simulink model "controllerJohnny"  (R2025b)
settings: Solver=ode45  StartTime=0.0  StopTime=15  RelTol=1e-3
values from neighbouring files (symbols this model uses):
  Ts = 0.01    [main.m]
settings Model: Creator=User  LastModifiedBy=User

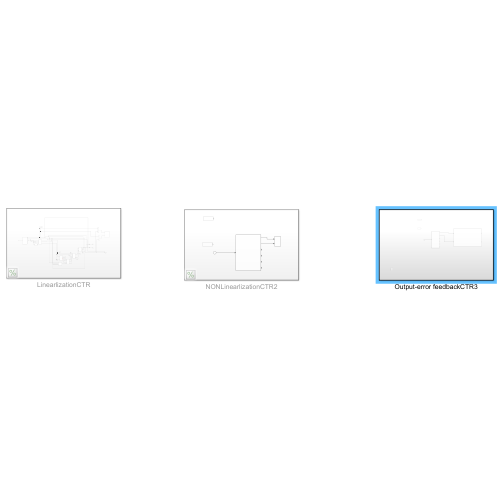
[thumbnail: Simulink's stored preview of the top-level diagram]
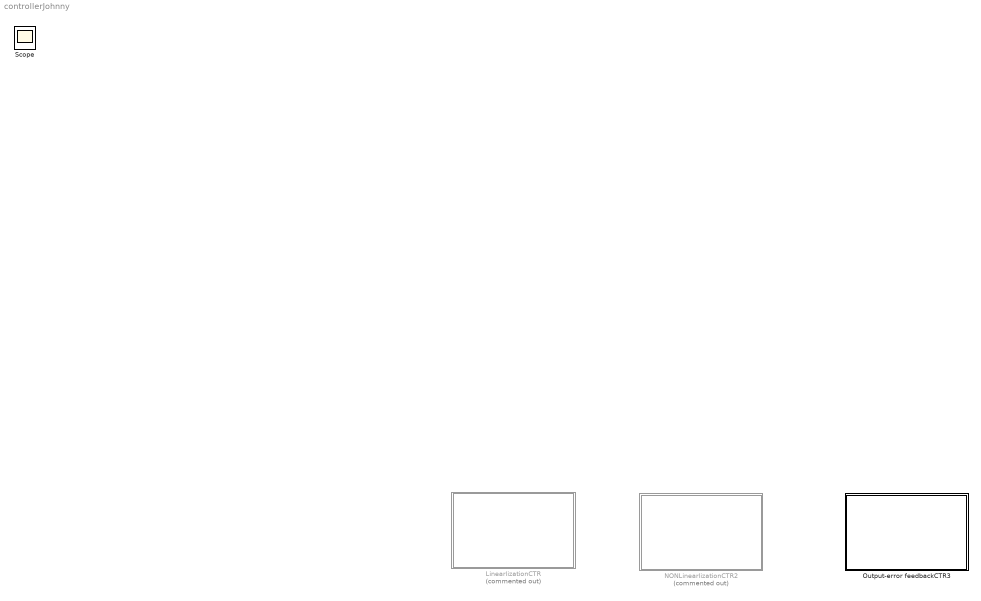
== system controllerJohnny ==
  LinearlizationCTR : Subsystem  Commented=on
  NONLinearlizationCTR2 : Subsystem  Commented=on
  Output-error feedbackCTR3 : Subsystem
  Scope : Scope
      settings: DataLoggingVariableName=ScopeData15

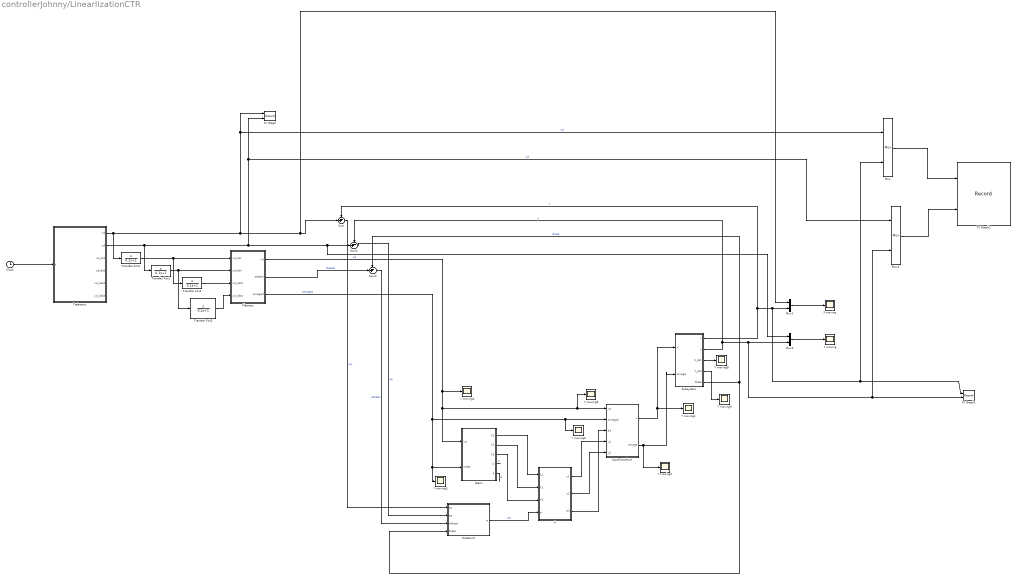
== system controllerJohnny/LinearlizationCTR ==
  Clock : Clock
  Flatness : MATLAB Function  TreatAsAtomicUnit=on
  Gians : MATLAB Function  TreatAsAtomicUnit=on
  InputTransform : MATLAB Function  TreatAsAtomicUnit=on
  Mux{,1,3..4} (4 alike) : Mux  Inputs=2
  Rotation1 : MATLAB Function  TreatAsAtomicUnit=on
  Subsystem : Subsystem
  Sum : Sum  Inputs=-+|
  Sum1 : Sum  Inputs=-+|
  Sum2 : Sum  Inputs=-+|
  Trajectory : MATLAB Function  TreatAsAtomicUnit=on
  Transfer Fcn{1..4} (4 alike) : TransferFcn  Numerator=[1 0]  Denominator=[0.1 1]
  U : MATLAB Function  TreatAsAtomicUnit=on
  X moving : Scope
      settings: ActiveDisplayYMinimum=-7.5707248352770318  ActiveDisplayYMaximum=6.89936023828367  DataLoggingVariableName=ScopeData2
  XY Graph : Record  NumPorts=2.0  FileSettingsInternal="{\"entries\":[{\"content\":{\"excelSettings\":{\"content\":{},\"type\":\"Streamout.ExcelSettings\"},\"parquetSettings\":{\"content\":{},\"type\":\"Streamout.ParquetSettings\"}},\"type\":\"Streamout.FileSettingStorage\",\"uuid\":\"\"}],\"packageUris\":[\"http:\\/\\/schema.mathworks.com\\/mf0\\/streamout_blocks\\/R2020a\"],\"version\":\"1.0\"}"  FrameSettings=[0, 0]  Layout=[1 1]  SignalsInternal="{\"entries\":[{\"content\":{},\"type\":\"RecordBlkView.InputSignals\",\"uuid\":\"\"}],\"packageUris\":[\"http:\\/\\/schema.mathworks.com\\/mf0\\/streamout_blocks\\/R2020a\"],\"version\":\"1.0\"}"  VisualizationBindings="{\"xyplotplugin\":{\"info\":[{\"series\":[],\"subplotID\":1}]}}"  CompatibilityTag=XY
  XY Graph1 : Record  NumPorts=2.0  FileSettingsInternal="{\"entries\":[{\"content\":{\"excelSettings\":{\"content\":{},\"type\":\"Streamout.ExcelSettings\"},\"parquetSettings\":{\"content\":{},\"type\":\"Streamout.ParquetSettings\"}},\"type\":\"Streamout.FileSettingStorage\",\"uuid\":\"\"}],\"packageUris\":[\"http:\\/\\/schema.mathworks.com\\/mf0\\/streamout_blocks\\/R2020a\"],\"version\":\"1.0\"}"  FrameSettings=[0, 0]  Layout=[1 1]  SignalsInternal="{\"entries\":[{\"content\":{},\"type\":\"RecordBlkView.InputSignals\",\"uuid\":\"\"}],\"packageUris\":[\"http:\\/\\/schema.mathworks.com\\/mf0\\/streamout_blocks\\/R2020a\"],\"version\":\"1.0\"}"  VisualizationBindings="{\"xyplotplugin\":{\"info\":[{\"series\":[],\"subplotID\":1}]}}"  CompatibilityTag=XY
  XY Graph2 : Record  NumPorts=2.0  FileSettingsInternal="{\"entries\":[{\"content\":{\"excelSettings\":{\"content\":{},\"type\":\"Streamout.ExcelSettings\"},\"parquetSettings\":{\"content\":{},\"type\":\"Streamout.ParquetSettings\"}},\"type\":\"Streamout.FileSettingStorage\",\"uuid\":\"\"}],\"packageUris\":[\"http:\\/\\/schema.mathworks.com\\/mf0\\/streamout_blocks\\/R2020a\"],\"version\":\"1.0\"}"  FrameSettings=[0, 0]  Layout=[1 1]  SignalsInternal="{\"entries\":[{\"content\":{\"signals\":[{\"content\":{\"blockPath\":[],\"dimensions\":[1],\"domain\":\"\",\"lineColor\":\"#ff6929\",\"lineWidth\":2,\"port\":1,\"signalID\":1,\"signalName\":\"Mux\"},\"type\":\"RecordBlkView.Signal\",\"uuid\":\"\"},{\"content\":{\"blockPath\":[],\"dimensions\":[1],\"domain\":\"\",\"lineColor\":\"#b746ff\",\"lineWidth\":2,\"port\":2,\"signalID\":2,\"signalName\":\"Mux4\"},\"type\":\"RecordBlkView.Signal\",\"uuid\":\"\"}]},\"type\":\"RecordBlkView.InputSignals\",\"uuid\":\"\"}],\"packageUris\":[\"http:\\/\\/schema.mathworks.com\\/mf0\\/streamout_blocks\\/R2020a\"],\"version\":\"1.0\"}"  VisualizationBindings="{\"xyplotplugin\":{\"info\":[{\"series\":[],\"subplotID\":1}]}}"  CompatibilityTag=XY
  Y moving{,1..6,8..9} (9 alike) : Scope
      Y moving settings: ActiveDisplayYMinimum=-5.0263813296916764  ActiveDisplayYMaximum=5.2374840982446349  DataLoggingVariableName=ScopeData3
      Y moving1 settings: ActiveDisplayYMinimum=-34.324914712581226  ActiveDisplayYMaximum=308.9242324132311  DataLoggingVariableName=ScopeData4
      Y moving2 settings: ActiveDisplayYMinimum=-1.6157130196688239E+7  ActiveDisplayYMaximum=1.4491472238781191E+7  DataLoggingVariableName=ScopeData5
      Y moving3 settings: ActiveDisplayYMinimum=4.999999999999944  ActiveDisplayYMaximum=5.0000000000000542  DataLoggingVariableName=ScopeData6
      Y moving4 settings: ActiveDisplayYMinimum=9.9999999999999982  ActiveDisplayYMaximum=10.000000000000002  DataLoggingVariableName=ScopeData7
      Y moving5 settings: ActiveDisplayYMinimum=0.99999999999999978  ActiveDisplayYMaximum=1  DataLoggingVariableName=ScopeData8
      Y moving6 settings: ActiveDisplayYMinimum=0.4  ActiveDisplayYMaximum=0.60000000000000009  DataLoggingVariableName=ScopeData9
      Y moving8 settings: ActiveDisplayYMinimum=-4.8047106790322678  ActiveDisplayYMaximum=12.533856742114697  DataLoggingVariableName=ScopeData11
      Y moving9 settings: ActiveDisplayYMinimum=-3.6998487914435718  ActiveDisplayYMaximum=4.6099967599268465  DataLoggingVariableName=ScopeData12
  wires:
  Subsystem/1(x) -> Mux/2, XY Graph1/1, Mux1/2, Sum/1  "x"
  Subsystem/5(theta) -> Rotation1/4(theta), Sum2/1  "theta"
  Trajectory/1(xd) -> Transfer Fcn4/1, Mux/1, XY Graph/1, Mux1/1, Sum/2  "xd"
  Flatness/3(omegad) -> Y moving3/1, Gians/2(wdes), Y moving6/1, InputTransform/2(omegad)  "omegad"
  Sum2/1 -> Rotation1/3(etheta)  "etheta"
  Gians/2(k2) -> U/2(k2)
  Sum/1 -> Rotation1/1(ex)  "ex"
  InputTransform/2(omega) -> Y moving2/1, Subsystem/2(omega)
  U/3(e3) -> InputTransform/3(e3)
  InputTransform/1(v) -> Subsystem/1(V), Y moving1/1
  Rotation1/1(e) -> U/4(e)  "ew"
  Gians/3(k3) -> U/3(k3)
  Gians/1(k1) -> U/1(k1)
  Flatness/1(vd) -> Y moving4/1, Gians/1(vd), Y moving5/1, InputTransform/1(vd)  "vd"
  Mux3/1 -> Y moving/1
  Subsystem/4(Y_dot) -> Y moving9/1
  Flatness/2(thetad) -> Sum2/2  "thetad"
  Subsystem/2(y) -> Mux4/2, XY Graph1/2, Mux3/2, Sum1/1  "y"
  Mux1/1 -> X moving/1
  U/1(u1) -> InputTransform/4(u1)
  Clock/1 -> Trajectory/1(t)
  Subsystem/3(X_dot) -> Y moving8/1
  U/2(u2) -> InputTransform/5(u2)
  Sum1/1 -> Rotation1/2(ey)  "ey"
  Mux4/1 -> XY Graph2/2
  Mux/1 -> XY Graph2/1
  Trajectory/2(yd) -> Transfer Fcn1/1, Mux4/1, XY Graph/2, Mux3/1, Sum1/2  "yd"
  Transfer Fcn4/1 -> Transfer Fcn2/1, Flatness/1(xd_dot)
  Transfer Fcn1/1 -> Flatness/2(yd_dot), Transfer Fcn3/1
  Transfer Fcn2/1 -> Flatness/3(xd_ddot)
  Transfer Fcn3/1 -> Flatness/4(yd_ddot)
  Gians/5(a) -> ?  "a"
  Gians/4(xi) -> ?  "xi"

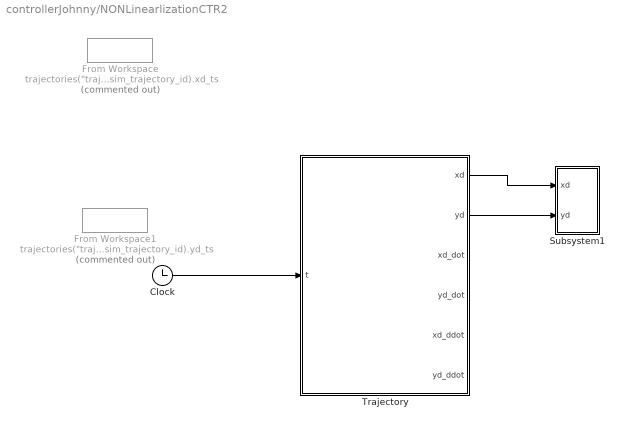
== system controllerJohnny/NONLinearlizationCTR2 ==
  Clock : Clock
  From Workspace : FromWorkspace  Commented=on  VariableName="trajectories(\"trajectory\"+sim_trajectory_id).xd_ts"  SampleTime=Ts  OutputAfterFinalValue=Holding final value
  From Workspace1 : FromWorkspace  Commented=on  VariableName="trajectories(\"trajectory\"+sim_trajectory_id).yd_ts"  SampleTime=Ts  OutputAfterFinalValue=Holding final value
  Subsystem1 : Subsystem
  Trajectory : MATLAB Function  TreatAsAtomicUnit=on
  wires:
  Clock/1 -> Trajectory/1(t)
  Trajectory/2(yd) -> Subsystem1/2(yd)
  Trajectory/1(xd) -> Subsystem1/1(xd)

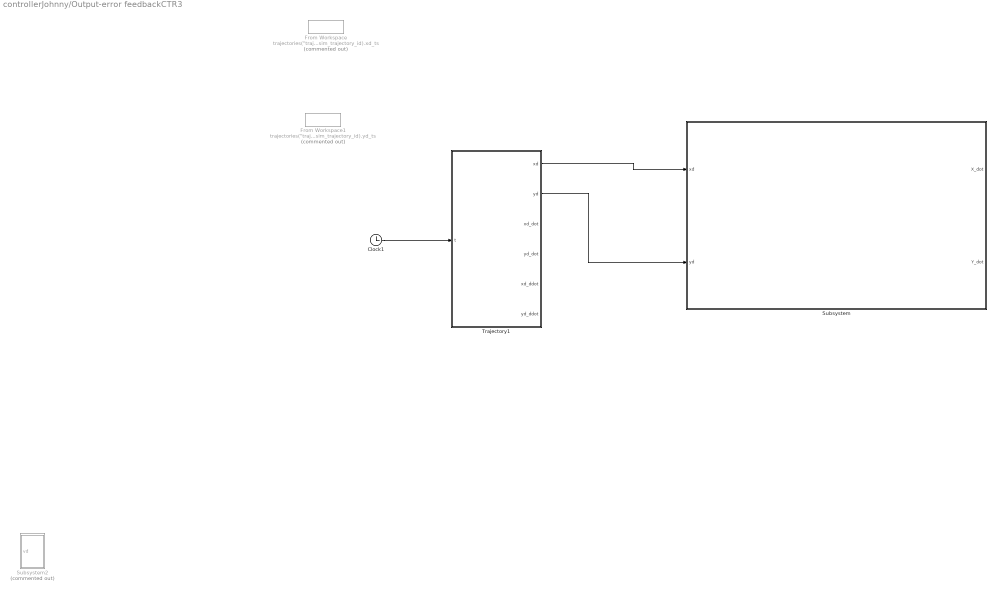
== system controllerJohnny/Output-error feedbackCTR3 ==
  Clock1 : Clock
  From Workspace : FromWorkspace  Commented=on  VariableName="trajectories(\"trajectory\"+sim_trajectory_id).xd_ts"  SampleTime=Ts  OutputAfterFinalValue=Holding final value
  From Workspace1 : FromWorkspace  Commented=on  VariableName="trajectories(\"trajectory\"+sim_trajectory_id).yd_ts"  SampleTime=Ts  OutputAfterFinalValue=Holding final value
  Subsystem : Subsystem
  Subsystem2 : Subsystem  Commented=on
  Trajectory1 : MATLAB Function  TreatAsAtomicUnit=on
  wires:
  Clock1/1 -> Trajectory1/1(t)
  Trajectory1/1(xd) -> Subsystem/1(xd)
  Trajectory1/2(yd) -> Subsystem/2(yd)

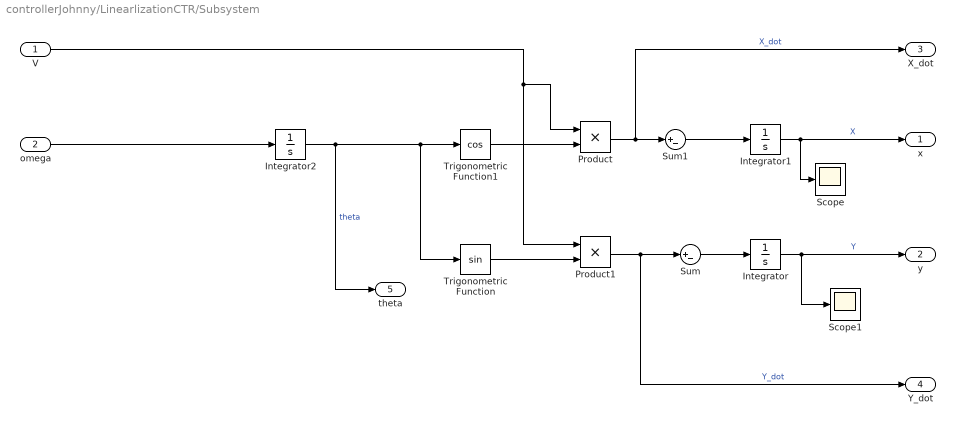
== system controllerJohnny/LinearlizationCTR/Subsystem ==
  V : Inport
  omega : Inport  Port=2
  Integrator : Integrator
  Integrator1 : Integrator
  Integrator2 : Integrator
  Product : Product
  Product1 : Product
  Scope : Scope
      settings: ActiveDisplayYMinimum=-0.63591257102151144  ActiveDisplayYMaximum=2.8001536498931303
  Scope1 : Scope
      settings: ActiveDisplayYMinimum=-1.1667967618896729  ActiveDisplayYMaximum=3.6680934698341847
  Sum : Sum  Inputs=|+-
  Sum1 : Sum  Inputs=|+-
  Trigonometric Function : Trigonometry
  Trigonometric Function1 : Trigonometry  Operator=cos
  x : Outport
  y : Outport  Port=2
  X_dot : Outport  Port=3
  Y_dot : Outport  Port=4
  theta : Outport  Port=5
  wires:
  Integrator/1 -> Scope1/1, y/1  "Y"
  Integrator2/1 -> theta/1, Trigonometric Function/1, Trigonometric Function1/1  "theta"
  Sum/1 -> Integrator/1
  V/1 -> Product/1, Product1/1
  Trigonometric Function1/1 -> Product/2
  Sum1/1 -> Integrator1/1
  Product/1 -> X_dot/1, Sum1/1  "X_dot"
  Integrator1/1 -> Scope/1, x/1  "X"
  Product1/1 -> Y_dot/1, Sum/1  "Y_dot"
  Trigonometric Function/1 -> Product1/2
  omega/1 -> Integrator2/1

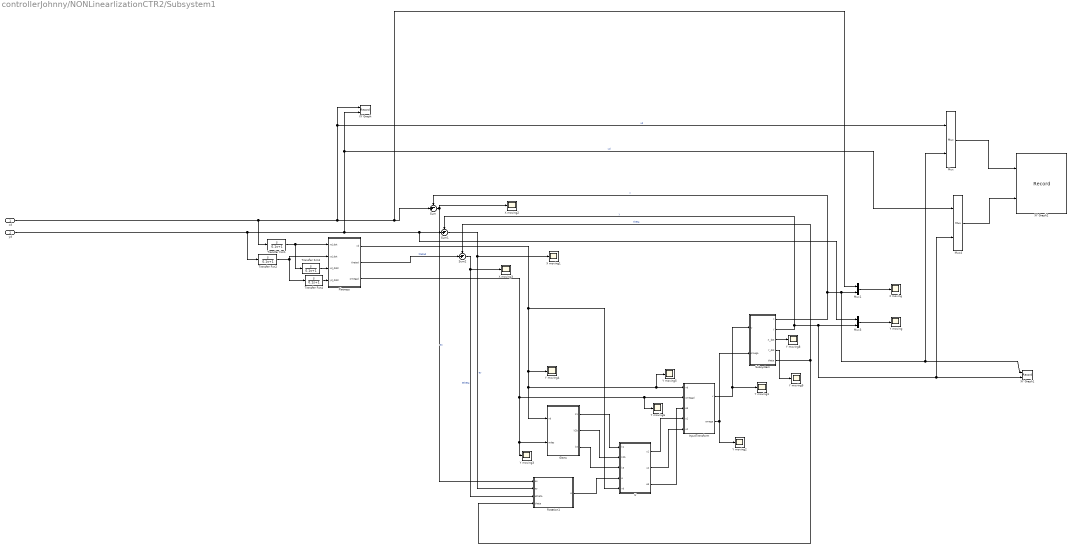
== system controllerJohnny/NONLinearlizationCTR2/Subsystem1 ==
  xd : Inport
  yd : Inport  Port=2
  Flatness : MATLAB Function  TreatAsAtomicUnit=on
  Gians : MATLAB Function  TreatAsAtomicUnit=on
  InputTransform : MATLAB Function  TreatAsAtomicUnit=on
  Mux{,1,3..4} (4 alike) : Mux  Inputs=2
  Rotation1 : MATLAB Function  TreatAsAtomicUnit=on
  Subsystem : Subsystem
  Sum : Sum  Inputs=-+|
  Sum1 : Sum  Inputs=-+|
  Sum2 : Sum  Inputs=-+|
  Transfer Fcn{1..4} (4 alike) : TransferFcn  Numerator=[1 0]  Denominator=[0.1 1]
  U : MATLAB Function  TreatAsAtomicUnit=on
  X moving{,1..3} (4 alike) : Scope
      X moving settings: ActiveDisplayYMinimum=-363.26549927941852  ActiveDisplayYMaximum=-359.6142263759865  DataLoggingVariableName=ScopeData2
      X moving1 settings: ActiveDisplayYMinimum=-1.8783922722321265  ActiveDisplayYMaximum=1.6589955287132554  DataLoggingVariableName=ScopeData10
      X moving2 settings: ActiveDisplayYMinimum=-3.0823097685833254  ActiveDisplayYMaximum=2.0935592914317827  DataLoggingVariableName=ScopeData13
      X moving3 settings: ActiveDisplayYMinimum=-3.3439097799700566  ActiveDisplayYMaximum=4.453783260307695  DataLoggingVariableName=ScopeData14
  XY Graph : Record  NumPorts=2.0  FileSettingsInternal="{\"entries\":[{\"content\":{\"excelSettings\":{\"content\":{},\"type\":\"Streamout.ExcelSettings\"},\"parquetSettings\":{\"content\":{},\"type\":\"Streamout.ParquetSettings\"}},\"type\":\"Streamout.FileSettingStorage\",\"uuid\":\"\"}],\"packageUris\":[\"http:\\/\\/schema.mathworks.com\\/mf0\\/streamout_blocks\\/R2020a\"],\"version\":\"1.0\"}"  FrameSettings=[0, 0]  Layout=[1 1]  SignalsInternal="{\"entries\":[{\"content\":{\"signals\":[{\"content\":{\"blockPath\":[],\"dimensions\":[1],\"domain\":\"\",\"lineColor\":\"#ff13a6\",\"lineWidth\":2,\"port\":1,\"signalID\":1,\"signalName\":\"xd\"},\"type\":\"RecordBlkView.Signal\",\"uuid\":\"\"},{\"content\":{\"blockPath\":[],\"dimensions\":[1],\"domain\":\"\",\"lineColor\":\"#fe330a\",\"lineWidth\":2,\"port\":2,\"signalID\":2,\"signalName\":\"yd\"},\"type\":\"RecordBlkView.Signal\",\"uuid\":\"\"}]},\"type\":\"RecordBlkView.InputSignals\",\"uuid\":\"\"}],\"packageUris\":[\"http:\\/\\/schema.mathworks.com\\/mf0\\/streamout_blocks\\/R2020a\"],\"version\":\"1.0\"}"  VisualizationBindings="{\"xyplotplugin\":{\"info\":[{\"series\":[],\"subplotID\":1}]}}"  CompatibilityTag=XY
  XY Graph1 : Record  NumPorts=2.0  FileSettingsInternal="{\"entries\":[{\"content\":{\"excelSettings\":{\"content\":{},\"type\":\"Streamout.ExcelSettings\"},\"parquetSettings\":{\"content\":{},\"type\":\"Streamout.ParquetSettings\"}},\"type\":\"Streamout.FileSettingStorage\",\"uuid\":\"\"}],\"packageUris\":[\"http:\\/\\/schema.mathworks.com\\/mf0\\/streamout_blocks\\/R2020a\"],\"version\":\"1.0\"}"  FrameSettings=[0, 0]  Layout=[1 1]  SignalsInternal="{\"entries\":[{\"content\":{\"signals\":[{\"content\":{\"blockPath\":[],\"dimensions\":[1],\"domain\":\"\",\"lineColor\":\"#22b573\",\"lineWidth\":2,\"port\":1,\"signalID\":1,\"signalName\":\"x\"},\"type\":\"RecordBlkView.Signal\",\"uuid\":\"\"},{\"content\":{\"blockPath\":[],\"dimensions\":[1],\"domain\":\"\",\"lineColor\":\"#0072bd\",\"lineWidth\":2,\"port\":2,\"signalID\":2,\"signalName\":\"y\"},\"type\":\"RecordBlkView.Signal\",\"uuid\":\"\"}]},\"type\":\"RecordBlkView.InputSignals\",\"uuid\":\"\"}],\"packageUris\":[\"http:\\/\\/schema.mathworks.com\\/mf0\\/streamout_blocks\\/R2020a\"],\"version\":\"1.0\"}"  VisualizationBindings="{\"xyplotplugin\":{\"info\":[{\"series\":[],\"subplotID\":1}]}}"  CompatibilityTag=XY
  XY Graph2 : Record  NumPorts=2.0  FileSettingsInternal="{\"entries\":[{\"content\":{\"excelSettings\":{\"content\":{},\"type\":\"Streamout.ExcelSettings\"},\"parquetSettings\":{\"content\":{},\"type\":\"Streamout.ParquetSettings\"}},\"type\":\"Streamout.FileSettingStorage\",\"uuid\":\"\"}],\"packageUris\":[\"http:\\/\\/schema.mathworks.com\\/mf0\\/streamout_blocks\\/R2020a\"],\"version\":\"1.0\"}"  FrameSettings=[0, 0]  Layout=[1 1]  SignalsInternal="{\"entries\":[{\"content\":{\"signals\":[{\"content\":{\"blockPath\":[],\"dimensions\":[2],\"domain\":\"\",\"hasChildren\":true,\"lineColor\":\"#64d413\",\"lineWidth\":2,\"port\":1,\"signalID\":1,\"signalName\":\"Mux\"},\"type\":\"RecordBlkView.Signal\",\"uuid\":\"\"},{\"content\":{\"blockPath\":[],\"channel\":[1],\"dimensions\":[2],\"domain\":\"\",\"lineColor\":\"#edb120\",\"lineWidth\":2,\"parentID\":1,\"port\":1,\"signalID\":2,\"signalName\":\"Mux\"},\"type\":\"RecordBlkView.Signal\",\"uuid\":\"\"},{\"content\":{\"blockPath\":[],\"channel\":[2],\"dimensions\":[2],\"domain\":\"\",\"lineColor\":\"#4dbeee\",\"lineWidth\":2,\"parentID\":1,\"port\":1,\"signalID\":3,\"signalName\":\"Mux\"},\"type\":\"RecordBlkView.Signal\",\"uuid\":\"\"},{\"content\":{\"blockPath\":[],\"dimensions\":[2],\"domain\":\"\",\"hasChildren\":true,\"lineColor\":\"#fe330a\",\"lineWidth\":2,\"port\":2,\"signalID\":4,\"signalName\":\"Mux4\"},\"type\":\"RecordBlkView.Signal\",\"uuid\":\"\"},{\"content\":{\"blockPath\":[],\"channel\":[1],\"dimensions\":[2],\"domain\":\"\",\"lineColor\":\"#77ac30\",\"lineWidth\":2,\"parentID\":4,\"port\":2,\"signalID\":5,\"signalName\":\"Mux4\"},\"type\":\"RecordBlkView.Signal\",\"uuid\":\"\"},{\"content\":{\"blockPath\":[],\"channel\":[2],\"dimensions\":[2],\"domain\":\"\",\"lineColor\":\"#a2142f\",\"lineWidth\":2,\"parentID\":4,\"port\":2,\"signalID\":6,\"signalName\":\"Mux4\"},\"type\":\"RecordBlkView.Signal\",\"uuid\":\"\"}]},\"type\":\"RecordBlkView.InputSignals\",\"uuid\":\"\"}],\"packageUris\":[\"http:\\/\\/schema.mathworks.com\\/mf0\\/streamout_blocks\\/R2020a\"],\"version\":\"1.0\"}"  VisualizationBindings="{\"xyplotplugin\":{\"info\":[{\"series\":[],\"subplotID\":1}]}}"  CompatibilityTag=XY
  Y moving{,1..6,8..9} (9 alike) : Scope
      Y moving settings: ActiveDisplayYMinimum=-7.4999627279123162  ActiveDisplayYMaximum=7.4999958513257434  DataLoggingVariableName=ScopeData3
      Y moving1 settings: ActiveDisplayYMinimum=-34.324914712581226  ActiveDisplayYMaximum=308.9242324132311  DataLoggingVariableName=ScopeData4
      Y moving2 settings: ActiveDisplayYMinimum=-1.6157130196688239E+7  ActiveDisplayYMaximum=1.4491472238781191E+7  DataLoggingVariableName=ScopeData5
      Y moving3 settings: ActiveDisplayYMinimum=4.999999999999944  ActiveDisplayYMaximum=5.0000000000000542  DataLoggingVariableName=ScopeData6
      Y moving4 settings: ActiveDisplayYMinimum=9.9999999999999982  ActiveDisplayYMaximum=10.000000000000002  DataLoggingVariableName=ScopeData7
      Y moving5 settings: ActiveDisplayYMinimum=0.99999999999999978  ActiveDisplayYMaximum=1  DataLoggingVariableName=ScopeData8
      Y moving6 settings: ActiveDisplayYMinimum=0.4  ActiveDisplayYMaximum=0.60000000000000009  DataLoggingVariableName=ScopeData9
      Y moving8 settings: ActiveDisplayYMinimum=-4.8047106790322678  ActiveDisplayYMaximum=12.533856742114697  DataLoggingVariableName=ScopeData11
      Y moving9 settings: ActiveDisplayYMinimum=-3.6998487914435718  ActiveDisplayYMaximum=4.6099967599268465  DataLoggingVariableName=ScopeData12
  wires:
  InputTransform/2(omega) -> Subsystem/2(omega), Y moving2/1
  Flatness/1(vd) -> U/5(vd), InputTransform/1(vd), Y moving5/1, Gians/1(vd), Y moving4/1
  Subsystem/5(theta) -> Rotation1/4(theta), Sum2/1  "theta"
  U/1(u1) -> InputTransform/4(u1)
  Subsystem/2(y) -> Sum1/1, Mux3/2, XY Graph1/2, Mux4/2  "y"
  Transfer Fcn2/1 -> Transfer Fcn4/1, Flatness/2(yd_dot)
  Transfer Fcn1/1 -> Transfer Fcn3/1, Flatness/1(xd_dot)
  Subsystem/1(x) -> Sum/1, Mux1/2, XY Graph1/1, Mux/2  "x"
  xd/1 -> Transfer Fcn1/1, Sum/2, Mux1/1, XY Graph/1, Mux/1  "xd"
  InputTransform/1(v) -> Y moving1/1, Subsystem/1(V)
  Transfer Fcn4/1 -> Flatness/4(yd_ddot)
  Sum2/1 -> X moving3/1, Rotation1/3(etheta)  "etheta"
  U/2(u2) -> InputTransform/5(u2)
  Mux3/1 -> Y moving/1
  Gians/1(k1) -> U/1(k1)
  Mux4/1 -> XY Graph2/2
  Mux1/1 -> X moving/1
  Sum1/1 -> X moving1/1, Rotation1/2(ey)  "ey"
  Subsystem/4(Y_dot) -> Y moving9/1
  Rotation1/1(e) -> U/4(e)
  Flatness/3(omegad) -> InputTransform/2(omegad), Y moving6/1, Gians/2(wdes), Y moving3/1
  Mux/1 -> XY Graph2/1
  Flatness/2(thetad) -> Sum2/2  "thetad"
  Gians/2(k2b) -> U/2(k2b)
  Transfer Fcn3/1 -> Flatness/3(xd_ddot)
  Sum/1 -> Rotation1/1(ex), X moving2/1  "ex"
  yd/1 -> Transfer Fcn2/1, Sum1/2, Mux3/1, XY Graph/2, Mux4/1  "yd"
  U/3(e3) -> InputTransform/3(e3)
  Gians/3(k3) -> U/3(k3)
  Subsystem/3(X_dot) -> Y moving8/1

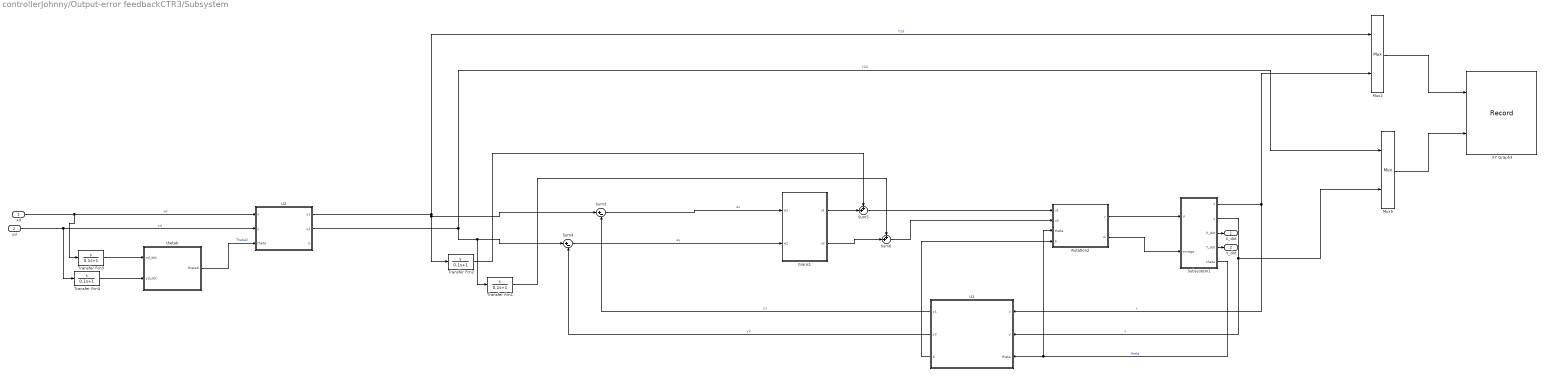
== system controllerJohnny/Output-error feedbackCTR3/Subsystem ==
  xd : Inport
  yd : Inport  Port=2
  Gians1 : MATLAB Function  TreatAsAtomicUnit=on
  Mux2 : Mux  Inputs=2
  Mux5 : Mux  Inputs=2
  Rotation2 : MATLAB Function  TreatAsAtomicUnit=on
  Subsystem1 : Subsystem
  Sum3 : Sum  Inputs=|+-
  Sum4 : Sum  Inputs=|+-
  Sum5 : Sum  Inputs=++|
  Sum6 : Sum  Inputs=++|
  Transfer Fcn{1..4} (4 alike) : TransferFcn  Numerator=[1 0]  Denominator=[0.1 1]
  U1 : MATLAB Function  TreatAsAtomicUnit=on
  U2 : MATLAB Function  TreatAsAtomicUnit=on
  XY Graph3 : Record  NumPorts=2.0  FileSettingsInternal="{\"entries\":[{\"content\":{\"excelSettings\":{\"content\":{},\"type\":\"Streamout.ExcelSettings\"},\"parquetSettings\":{\"content\":{},\"type\":\"Streamout.ParquetSettings\"}},\"type\":\"Streamout.FileSettingStorage\",\"uuid\":\"\"}],\"packageUris\":[\"http:\\/\\/schema.mathworks.com\\/mf0\\/streamout_blocks\\/R2020a\"],\"version\":\"1.0\"}"  FrameSettings=[0, 0]  Layout=[1 1]  SignalsInternal="{\"entries\":[{\"content\":{\"signals\":[{\"content\":{\"blockPath\":[],\"dimensions\":[2],\"domain\":\"\",\"hasChildren\":true,\"lineColor\":\"#4dbeee\",\"lineWidth\":2,\"port\":1,\"sid\":[\"\"],\"signalID\":1,\"signalName\":\"Mux2\"},\"type\":\"RecordBlkView.Signal\",\"uuid\":\"\"},{\"content\":{\"blockPath\":[],\"channel\":[1],\"dimensions\":[2],\"domain\":\"\",\"lineColor\":\"#139fff\",\"lineWidth\":2,\"parentID\":1,\"plots\":[ 1 ],\"port\":1,\"sid\":[\"\"],\"signalID\":2,\"signalName\":\"Mux2\"},\"type\":\"RecordBlkView.Signal\",\"uuid\":\"\"},{\"content\":{\"blockPath\":[],\"dimensions\":[2],\"domain\":\"\",\"hasChildren\":true,\"lineColor\":\"#139fff\",\"lineWidth\":2,\"port\":2,\"sid\":[\"\"],\"signalID\":3,\"signalName\":\"Mux5\"},\"type\":\"RecordBlkView.Signal\",\"uuid\":\"\"},{\"content\":{\"blockPath\":[],\"channel\":[1],\"dimensions\":[2],\"domain\":\"\",\"lineColor\":\"#139fff\",\"lineWidth\":2,\"parentID\":3,\"plots\":[ 1 ],\"port\":2,\"sid\":[\"\"],\"signalID\":4,\"signalName\":\"Mux5\"},\"type\":\"RecordBlkView.Signal\",\"uuid\":\"\"},{\"content\":{\"blockPath\":[],\"channel\":[2],\"dimensions\":[2],\"domain\":\"\",\"lineColor\":\"#fe330a\",\"lineWidth\":2,\"parentID\":1,\"plots\":[ 1 ],\"port\":1,\"sid\":[\"\"],\"signalID\":5,\"signalName\":\"Mux2\"},\"type\":\"RecordBlkView.Signal\",\"uuid\":\"\"},{\"content\":{\"blockPath\":[],\"channel\":[2],\"dimensions\":[2],\"domain\":\"\",\"lineColor\":\"#fe330a\",\"lineWidth\":2,\"parentID\":3,\"plots\":[ 1 ],\"port\":2,\"sid\":[\"\"],\"signalID\":6,\"signalName\":\"Mux5\"},\"type\":\"RecordBlkView.Signal\",\"uuid\":\"\"}]},\"type\":\"RecordBlkView.InputSignals\",\"uuid\":\"\"}],\"packageUris\":[\"http:\\/\\/schema.mathworks.com\\/mf0\\/streamout_blocks\\/R2020a\"],\"version\":\"1.0\"}"  VisualizationBindings="{\"xyplotplugin\":{\"info\":[{\"series\":[{\"bindingParametersList\":[{\"parameter\":\"X-Axis\",\"signalID\":2,\"signalName\":\"Mux2(1)\"},{\"parameter\":\"Y-Axis\",\"signalID\":4,\"signalName\":\"Mux5(1)\"}],\"seriesID\":0},{\"bindingParametersList\":[{\"parameter\":\"X-Axis\",\"signalID\":5,\"signalName\":\"Mux2(2)\"},{\"parameter\":\"Y-Axis\",\"signalID\":6,\"signalName\":\"Mux5(2)\"}],\"seriesID\":1}],\"subplotID\":1}]}}"  CompatibilityTag=XY
  thetab : MATLAB Function  TreatAsAtomicUnit=on
  X_dot : Outport
  Y_dot : Outport  Port=2
  wires:
  Sum3/1 -> Gians1/1(e1)  "ex"
  Gians1/2(u2) -> Sum6/2
  U2/2(y2) -> Transfer Fcn1/1, Sum4/1, Mux5/1  "Y2d"
  Subsystem1/2(y) -> Mux5/2, U1/2(y)  "y"
  Mux2/1 -> XY Graph3/1
  Sum6/1 -> Rotation2/2(u2)
  Transfer Fcn2/1 -> Sum5/1
  Mux5/1 -> XY Graph3/2
  U1/2(y2) -> Sum4/2  "y2"
  Rotation2/1(v) -> Subsystem1/1(V)
  Sum4/1 -> Gians1/2(e2)  "ey"
  Sum5/1 -> Rotation2/1(u1)
  Subsystem1/4(Y_dot) -> Y_dot/1
  Gians1/1(u1) -> Sum5/2
  U2/1(y1) -> Transfer Fcn2/1, Sum3/1, Mux2/1  "Y1d"
  Subsystem1/1(x) -> U1/1(x), Mux2/2  "x"
  Rotation2/2(w) -> Subsystem1/2(omega)
  U1/3(b) -> Rotation2/4(b)
  U1/1(y1) -> Sum3/2  "y1"
  Transfer Fcn1/1 -> Sum6/1
  Subsystem1/3(X_dot) -> X_dot/1
  yd/1 -> Transfer Fcn4/1, U2/2(y)  "yd"
  xd/1 -> Transfer Fcn3/1, U2/1(x)  "xd"
  Transfer Fcn3/1 -> thetab/1(xd_dot)
  Transfer Fcn4/1 -> thetab/2(yd_dot)
  Subsystem1/5(theta) -> Rotation2/3(theta), U1/3(theta)  "theta"
  thetab/1(thetab) -> U2/3(theta)  "ThetaD"

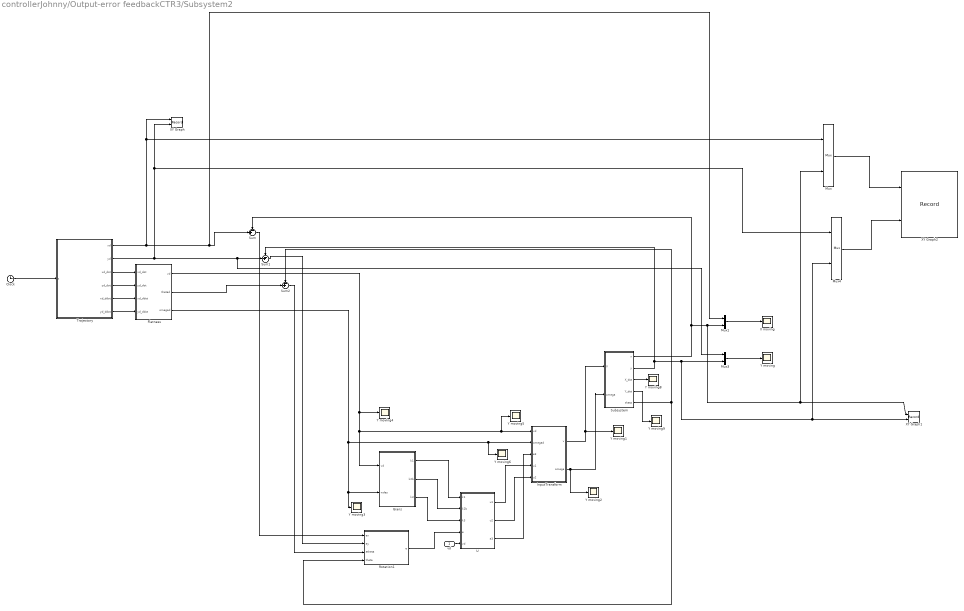
== system controllerJohnny/Output-error feedbackCTR3/Subsystem2 ==
  vd : Inport
  Clock : Clock
  Flatness : MATLAB Function  TreatAsAtomicUnit=on
  Gians : MATLAB Function  TreatAsAtomicUnit=on
  InputTransform : MATLAB Function  TreatAsAtomicUnit=on
  Mux{,1,3..4} (4 alike) : Mux  Inputs=2
  Rotation1 : MATLAB Function  TreatAsAtomicUnit=on
  Subsystem : Subsystem
  Sum : Sum  Inputs=-+|
  Sum1 : Sum  Inputs=-+|
  Sum2 : Sum  Inputs=-+|
  Trajectory : MATLAB Function  TreatAsAtomicUnit=on
  U : MATLAB Function  TreatAsAtomicUnit=on
  X moving : Scope
      settings: ActiveDisplayYMinimum=-7.5707248352770318  ActiveDisplayYMaximum=6.89936023828367  DataLoggingVariableName=ScopeData2
  XY Graph : Record  NumPorts=2.0  FileSettingsInternal="{\"entries\":[{\"content\":{\"excelSettings\":{\"content\":{},\"type\":\"Streamout.ExcelSettings\"},\"parquetSettings\":{\"content\":{},\"type\":\"Streamout.ParquetSettings\"}},\"type\":\"Streamout.FileSettingStorage\",\"uuid\":\"\"}],\"packageUris\":[\"http:\\/\\/schema.mathworks.com\\/mf0\\/streamout_blocks\\/R2020a\"],\"version\":\"1.0\"}"  FrameSettings=[0, 0]  Layout=[1 1]  SignalsInternal="{\"entries\":[{\"content\":{},\"type\":\"RecordBlkView.InputSignals\",\"uuid\":\"\"}],\"packageUris\":[\"http:\\/\\/schema.mathworks.com\\/mf0\\/streamout_blocks\\/R2020a\"],\"version\":\"1.0\"}"  VisualizationBindings="{\"xyplotplugin\":{\"info\":[{\"series\":[],\"subplotID\":1}]}}"  CompatibilityTag=XY
  XY Graph1 : Record  NumPorts=2.0  FileSettingsInternal="{\"entries\":[{\"content\":{\"excelSettings\":{\"content\":{},\"type\":\"Streamout.ExcelSettings\"},\"parquetSettings\":{\"content\":{},\"type\":\"Streamout.ParquetSettings\"}},\"type\":\"Streamout.FileSettingStorage\",\"uuid\":\"\"}],\"packageUris\":[\"http:\\/\\/schema.mathworks.com\\/mf0\\/streamout_blocks\\/R2020a\"],\"version\":\"1.0\"}"  FrameSettings=[0, 0]  Layout=[1 1]  SignalsInternal="{\"entries\":[{\"content\":{},\"type\":\"RecordBlkView.InputSignals\",\"uuid\":\"\"}],\"packageUris\":[\"http:\\/\\/schema.mathworks.com\\/mf0\\/streamout_blocks\\/R2020a\"],\"version\":\"1.0\"}"  VisualizationBindings="{\"xyplotplugin\":{\"info\":[{\"series\":[],\"subplotID\":1}]}}"  CompatibilityTag=XY
  XY Graph2 : Record  NumPorts=2.0  FileSettingsInternal="{\"entries\":[{\"content\":{\"excelSettings\":{\"content\":{},\"type\":\"Streamout.ExcelSettings\"},\"parquetSettings\":{\"content\":{},\"type\":\"Streamout.ParquetSettings\"}},\"type\":\"Streamout.FileSettingStorage\",\"uuid\":\"\"}],\"packageUris\":[\"http:\\/\\/schema.mathworks.com\\/mf0\\/streamout_blocks\\/R2020a\"],\"version\":\"1.0\"}"  FrameSettings=[0, 0]  Layout=[1 1]  SignalsInternal="{\"entries\":[{\"content\":{},\"type\":\"RecordBlkView.InputSignals\",\"uuid\":\"\"}],\"packageUris\":[\"http:\\/\\/schema.mathworks.com\\/mf0\\/streamout_blocks\\/R2020a\"],\"version\":\"1.0\"}"  VisualizationBindings="{\"xyplotplugin\":{\"info\":[{\"series\":[],\"subplotID\":1}]}}"  CompatibilityTag=XY
  Y moving{,1..6,8..9} (9 alike) : Scope
      Y moving settings: ActiveDisplayYMinimum=-7.4999627279123162  ActiveDisplayYMaximum=7.4999958513257434  DataLoggingVariableName=ScopeData3
      Y moving1 settings: ActiveDisplayYMinimum=-34.324914712581226  ActiveDisplayYMaximum=308.9242324132311  DataLoggingVariableName=ScopeData4
      Y moving2 settings: ActiveDisplayYMinimum=-1.6157130196688239E+7  ActiveDisplayYMaximum=1.4491472238781191E+7  DataLoggingVariableName=ScopeData5
      Y moving3 settings: ActiveDisplayYMinimum=4.999999999999944  ActiveDisplayYMaximum=5.0000000000000542  DataLoggingVariableName=ScopeData6
      Y moving4 settings: ActiveDisplayYMinimum=9.9999999999999982  ActiveDisplayYMaximum=10.000000000000002  DataLoggingVariableName=ScopeData7
      Y moving5 settings: ActiveDisplayYMinimum=0.99999999999999978  ActiveDisplayYMaximum=1  DataLoggingVariableName=ScopeData8
      Y moving6 settings: ActiveDisplayYMinimum=0.4  ActiveDisplayYMaximum=0.60000000000000009  DataLoggingVariableName=ScopeData9
      Y moving8 settings: ActiveDisplayYMinimum=-4.8047106790322678  ActiveDisplayYMaximum=12.533856742114697  DataLoggingVariableName=ScopeData11
      Y moving9 settings: ActiveDisplayYMinimum=-3.6998487914435718  ActiveDisplayYMaximum=4.6099967599268465  DataLoggingVariableName=ScopeData12
  wires:
  Trajectory/3(xd_dot) -> Flatness/1(xd_dot)
  Mux3/1 -> Y moving/1
  Flatness/3(omegad) -> Y moving3/1, Gians/2(wdes), Y moving6/1, InputTransform/2(omegad)
  InputTransform/1(v) -> Subsystem/1(V), Y moving1/1
  Sum/1 -> Rotation1/1(ex)
  Subsystem/2(y) -> Mux4/2, XY Graph1/2, Mux3/2, Sum1/1
  Subsystem/1(x) -> Mux/2, XY Graph1/1, Mux1/2, Sum/1
  Trajectory/1(xd) -> Mux/1, XY Graph/1, Mux1/1, Sum/2
  Sum2/1 -> Rotation1/3(etheta)
  Trajectory/5(xd_ddot) -> Flatness/3(xd_ddot)
  Sum1/1 -> Rotation1/2(ey)
  Flatness/1(vd) -> Y moving4/1, Gians/1(vd), Y moving5/1, InputTransform/1(vd)
  Mux/1 -> XY Graph2/1
  Trajectory/2(yd) -> Mux4/1, XY Graph/2, Mux3/1, Sum1/2
  Trajectory/4(yd_dot) -> Flatness/2(yd_dot)
  Subsystem/3(X_dot) -> Y moving8/1
  Gians/1(k1) -> U/1(k1)
  Subsystem/5(theta) -> Rotation1/4(theta), Sum2/1
  Mux4/1 -> XY Graph2/2
  Gians/2(k2b) -> U/2(k2b)
  Rotation1/1(e) -> U/4(e)
  U/2(u2) -> InputTransform/5(u2)
  Subsystem/4(Y_dot) -> Y moving9/1
  InputTransform/2(omega) -> Y moving2/1, Subsystem/2(omega)
  Flatness/2(thetad) -> Sum2/2
  U/1(u1) -> InputTransform/4(u1)
  Clock/1 -> Trajectory/1(t)
  Mux1/1 -> X moving/1
  vd/1 -> U/5(vd)
  Trajectory/6(yd_ddot) -> Flatness/4(yd_ddot)
  U/3(e3) -> InputTransform/3(e3)
  Gians/3(k3) -> U/3(k3)

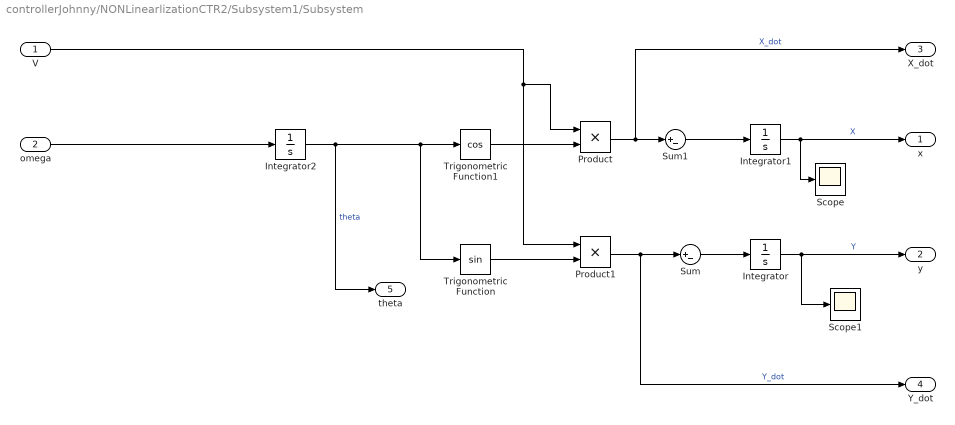
== system controllerJohnny/NONLinearlizationCTR2/Subsystem1/Subsystem ==
  V : Inport
  omega : Inport  Port=2
  Integrator : Integrator
  Integrator1 : Integrator
  Integrator2 : Integrator
  Product : Product
  Product1 : Product
  Scope : Scope
      settings: ActiveDisplayYMinimum=-0.63591257102151144  ActiveDisplayYMaximum=2.8001536498931303
  Scope1 : Scope
      settings: ActiveDisplayYMinimum=-1.1667967618896729  ActiveDisplayYMaximum=3.6680934698341847
  Sum : Sum  Inputs=|+-
  Sum1 : Sum  Inputs=|+-
  Trigonometric Function : Trigonometry
  Trigonometric Function1 : Trigonometry  Operator=cos
  x : Outport
  y : Outport  Port=2
  X_dot : Outport  Port=3
  Y_dot : Outport  Port=4
  theta : Outport  Port=5
  wires:
  omega/1 -> Integrator2/1
  Trigonometric Function/1 -> Product1/2
  Product1/1 -> Sum/1, Y_dot/1  "Y_dot"
  Integrator1/1 -> x/1, Scope/1  "X"
  Product/1 -> Sum1/1, X_dot/1  "X_dot"
  Sum1/1 -> Integrator1/1
  Trigonometric Function1/1 -> Product/2
  V/1 -> Product1/1, Product/1
  Sum/1 -> Integrator/1
  Integrator2/1 -> Trigonometric Function1/1, Trigonometric Function/1, theta/1  "theta"
  Integrator/1 -> y/1, Scope1/1  "Y"

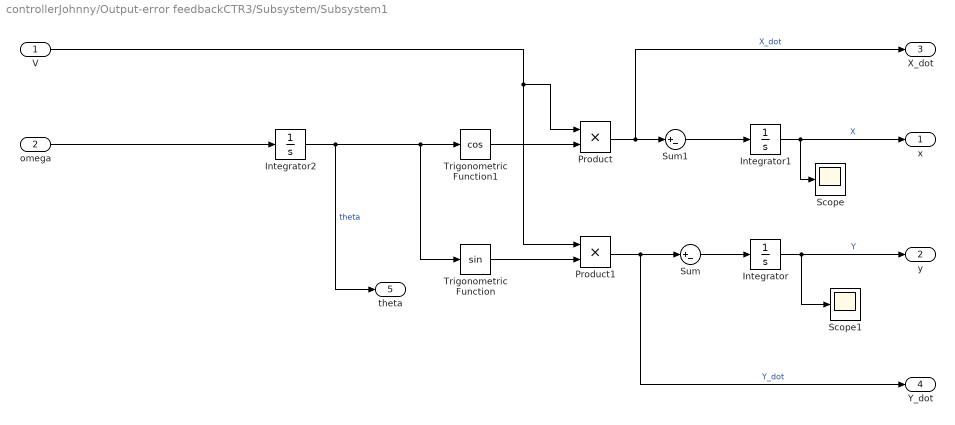
== system controllerJohnny/Output-error feedbackCTR3/Subsystem/Subsystem1 ==
  V : Inport
  omega : Inport  Port=2
  Integrator : Integrator
  Integrator1 : Integrator
  Integrator2 : Integrator
  Product : Product
  Product1 : Product
  Scope : Scope
      settings: ActiveDisplayYMinimum=-0.63591257102151144  ActiveDisplayYMaximum=2.8001536498931303
  Scope1 : Scope
      settings: ActiveDisplayYMinimum=-1.1667967618896729  ActiveDisplayYMaximum=3.6680934698341847
  Sum : Sum  Inputs=|+-
  Sum1 : Sum  Inputs=|+-
  Trigonometric Function : Trigonometry
  Trigonometric Function1 : Trigonometry  Operator=cos
  x : Outport
  y : Outport  Port=2
  X_dot : Outport  Port=3
  Y_dot : Outport  Port=4
  theta : Outport  Port=5
  wires:
  omega/1 -> Integrator2/1
  Trigonometric Function/1 -> Product1/2
  Product1/1 -> Sum/1, Y_dot/1  "Y_dot"
  Integrator1/1 -> x/1, Scope/1  "X"
  Product/1 -> Sum1/1, X_dot/1  "X_dot"
  Sum1/1 -> Integrator1/1
  Trigonometric Function1/1 -> Product/2
  V/1 -> Product1/1, Product/1
  Sum/1 -> Integrator/1
  Integrator2/1 -> Trigonometric Function1/1, Trigonometric Function/1, theta/1  "theta"
  Integrator/1 -> y/1, Scope1/1  "Y"

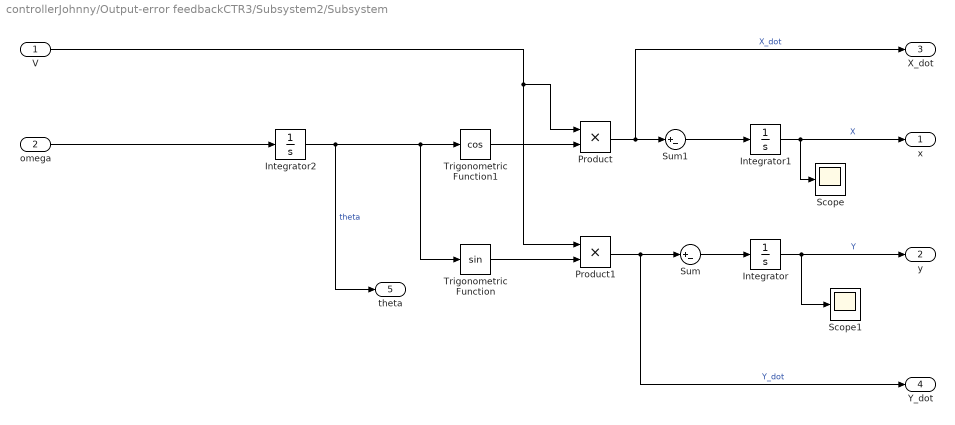
== system controllerJohnny/Output-error feedbackCTR3/Subsystem2/Subsystem ==
  V : Inport
  omega : Inport  Port=2
  Integrator : Integrator
  Integrator1 : Integrator
  Integrator2 : Integrator
  Product : Product
  Product1 : Product
  Scope : Scope
      settings: ActiveDisplayYMinimum=-0.63591257102151144  ActiveDisplayYMaximum=2.8001536498931303
  Scope1 : Scope
      settings: ActiveDisplayYMinimum=-1.1667967618896729  ActiveDisplayYMaximum=3.6680934698341847
  Sum : Sum  Inputs=|+-
  Sum1 : Sum  Inputs=|+-
  Trigonometric Function : Trigonometry
  Trigonometric Function1 : Trigonometry  Operator=cos
  x : Outport
  y : Outport  Port=2
  X_dot : Outport  Port=3
  Y_dot : Outport  Port=4
  theta : Outport  Port=5
  wires:
  Integrator/1 -> Scope1/1, y/1  "Y"
  Integrator2/1 -> theta/1, Trigonometric Function/1, Trigonometric Function1/1  "theta"
  Sum/1 -> Integrator/1
  V/1 -> Product/1, Product1/1
  Trigonometric Function1/1 -> Product/2
  Sum1/1 -> Integrator1/1
  Product/1 -> X_dot/1, Sum1/1  "X_dot"
  Integrator1/1 -> Scope/1, x/1  "X"
  Product1/1 -> Y_dot/1, Sum/1  "Y_dot"
  Trigonometric Function/1 -> Product1/2
  omega/1 -> Integrator2/1

== matlab function controllerJohnny/LinearlizationCTR/InputTransform ==
  data: vd input; omegad input; e3 input; u1 input; u2 input; v output; omega output
function [v, omega] = input_transform(vd, omegad, e3, u1, u2)

v     = vd*cos(e3) - u1;
omega = omegad - u2;

end

== matlab function controllerJohnny/NONLinearlizationCTR2/Subsystem1/Flatness ==
  data: xd_dot input; vd output; thetad output; omegad output; yd_dot input; xd_ddot input; yd_ddot input
function [vd, thetad, omegad] = flatness(xd_dot, yd_dot, xd_ddot, yd_ddot)

vd = sqrt(xd_dot^2 + yd_dot^2);
thetad = atan2(yd_dot, xd_dot);
omegad = (xd_dot*yd_ddot - yd_dot*xd_ddot)/max(vd^2,1e-3);
end

== matlab function controllerJohnny/NONLinearlizationCTR2/Subsystem1/Gians ==
  data: vd input; k1 output; k2b output; k3 output; wdes input
function [k1, k2b, k3 ] = gain_scheduler(vd, wdes)
% Implements Eq. (1.211)

xi = 0.7;
k2b = 100;
a = sqrt(k2b * vd + wdes^2);
k1 = 2*xi*a;
k3 = 2*xi*a;
        




end

== matlab function controllerJohnny/NONLinearlizationCTR2/Subsystem1/InputTransform ==
  data: vd input; omegad input; e3 input; u1 input; u2 input; v output; omega output
function [v, omega] = input_transform(vd, omegad, e3, u1, u2)

v     = vd*cos(e3) - u1;
omega = omegad - u2;

end

== matlab function controllerJohnny/NONLinearlizationCTR2/Subsystem1/Rotation1 ==
  data: ex input; e output; ey input; etheta input; theta input
function e = error_transform(ex, ey, etheta, theta)
theta = wrapTo2Pi(theta)
e1 =  ex*cos(theta) + ey*sin(theta);
e2 = -ex*sin(theta) + ey*cos(theta);
e3 = etheta;

e = [e1 e2 e3];
end

== matlab function controllerJohnny/NONLinearlizationCTR2/Trajectory ==
  data: t input; xd output; yd output; xd_dot output; yd_dot output; xd_ddot output; yd_ddot output
function [xd, yd, xd_dot, yd_dot, xd_ddot, yd_ddot] = traj(t)
R = 6;
w = 0.4;

xd = R*cos(w*t);
yd = R*sin(w*t);

xd_dot = -R*w*sin(w*t);
yd_dot =  R*w*cos(w*t);

xd_ddot = -R*w^2*cos(w*t);
yd_ddot = -R*w^2*sin(w*t);
end

%{ 

    T = mod(t,8);
    v = 2;

    if T < 2
                xd = v*T; yd = 0;
                xd_dot = v; yd_dot = 0;
            elseif T < 4
                xd = v*2; yd = v*(T-2);
                xd_dot = 0; yd_dot = v;
            elseif T < 6
                xd = v*(6-T); yd = v*2;
                xd_dot = -v; yd_dot = 0;
            else
                xd = 0; yd = v*(8-T);
                xd_dot = 0; yd_dot = -v;
    end

            xd_ddot = 0;
            yd_ddot = 0;
    end

%}

%{
% Square parameters
L = 18;        % side length [m]
v = 2;      % linear speed [m/s]
T = L / v;    % time per side

% Make trajectory periodic
t = mod(t, 4*T);

% Initialize outputs (VERY IMPORTANT for Simulink)
xd = 0; yd = 0;
xd_dot = 0; yd_dot = 0;
xd_ddot = 0; yd_ddot = 0;

% ---- Side 1: move right ----
if t < T
    xd = v*t;
    yd = 0;
    xd_dot = v;
    yd_dot = 0;

% ---- Side 2: move up ----
elseif t < 2*T
    xd = L;
    yd = v*(t - T);
    xd_dot = 0;
    yd_dot = v;

% ---- Side 3: move left ----
elseif t < 3*T
    xd = L - v*(t - 2*T);
    yd = L;
    xd_dot = -v;
    yd_dot = 0;

% ---- Side 4: move down ----
else
    xd = 0;
    yd = L - v*(t - 3*T);
    xd_dot = 0;
    yd_dot = -v;
end
end 
%}

== matlab function controllerJohnny/NONLinearlizationCTR2/Subsystem1/U ==
  data: k1 input; k2b input; k3 input; e input; u1 output; u2 output; e3 output; vd input
function [u1, u2,e3] = nonlinear_controller(k1, k2b, k3 ,e,vd)
e3 =e(3);
sinc_e3 = sin(e3) / (e3 + 1e-6);


u1 = -k1 * e(1);
u2 = -k2b * vd * sinc_e3 * e(2) - k3 * e3;


end

== matlab function controllerJohnny/Output-error feedbackCTR3/Subsystem/Rotation2 ==
  data: u1 input; v output; u2 input; theta input; w output; b input
function [v,w] = error_transform(u1, u2 , theta,b)

v = u1 * cos(theta)       + u2 * sin(theta);
w = u1 * (- sin(theta)/b) + u2 *cos(theta)/b;
end

== matlab function controllerJohnny/Output-error feedbackCTR3/Subsystem2/Flatness ==
  data: xd_dot input; vd output; thetad output; omegad output; yd_dot input; xd_ddot input; yd_ddot input
function [vd, thetad, omegad] = flatness(xd_dot, yd_dot, xd_ddot, yd_ddot)

vd = sqrt(xd_dot^2 + yd_dot^2);
thetad = atan2(yd_dot, xd_dot);
omegad = (xd_dot*yd_ddot - yd_dot*xd_ddot)/max(vd^2,1e-3);
end

== matlab function controllerJohnny/Output-error feedbackCTR3/Subsystem2/Gians ==
  data: vd input; k1 output; k2b output; k3 output; wdes input
function [k1, k2b, k3 ] = gain_scheduler(vd, wdes)
% Implements Eq. (1.211)

xi = 0.9;
k2b = 100;
a = sqrt(k2b * vd + wdes^2);
k1 = 2*xi*a;
k3 = 2*xi*a;
        




end

== matlab function controllerJohnny/Output-error feedbackCTR3/Subsystem2/InputTransform ==
  data: vd input; omegad input; e3 input; u1 input; u2 input; v output; omega output
function [v, omega] = input_transform(vd, omegad, e3, u1, u2)

v     = vd*cos(e3) - u1;
omega = omegad - u2;

end

== matlab function controllerJohnny/Output-error feedbackCTR3/Subsystem2/Rotation1 ==
  data: ex input; e output; ey input; etheta input; theta input
function e = error_transform(ex, ey, etheta, theta)

e1 =  ex*cos(theta) + ey*sin(theta);
e2 = -ex*sin(theta) + ey*cos(theta);
e3 = etheta;

e = [e1 e2 e3];
end

== matlab function controllerJohnny/Output-error feedbackCTR3/Subsystem2/Trajectory ==
  data: t input; xd output; yd output; xd_dot output; yd_dot output; xd_ddot output; yd_ddot output
function [xd, yd, xd_dot, yd_dot, xd_ddot, yd_ddot] = traj(t)
R = 6;
w = 0.4;

xd = R*cos(w*t);
yd = R*sin(w*t);

xd_dot = -R*w*sin(w*t);
yd_dot =  R*w*cos(w*t);

xd_ddot = -R*w^2*cos(w*t);
yd_ddot = -R*w^2*sin(w*t);
end

== matlab function controllerJohnny/Output-error feedbackCTR3/Subsystem2/U ==
  data: k1 input; k2b input; k3 input; e input; u1 output; u2 output; e3 output; vd input
function [u1, u2,e3] = nonlinear_controller(k1, k2b, k3 ,e,vd)
e3 =e(3);
sinc_e3 = sin(e3) / (e3 + 1e-6);
u1 = -k1 * e(1);
u2 = -k2b * e(2) - k3 * e(3);

u1 = -k1 * e(1);
u2 = -k2b * vd * sinc_e3 * e(2) - k3 * e3;
e3 =e(3);


end

== matlab function controllerJohnny/Output-error feedbackCTR3/Subsystem/Gians1 ==
  data: e1 input; u1 output; u2 output; e2 input
function [u1,u2 ] = gain_scheduler(e1,e2)

k1 = 2;
k2 = 2;

u1 = k1 * e1;
u2 = k2 * e2;



end

== matlab function controllerJohnny/Output-error feedbackCTR3/Subsystem/U1 ==
  data: x input; y input; theta input; y1 output; y2 output; b output
function [y1, y2,b] = inversTransform(x,y,theta)
b = 0.5;
y1 = x + b * cos(theta);
y2 = y + b * sin(theta);

end

== matlab function controllerJohnny/Output-error feedbackCTR3/Subsystem/thetab ==
  data: xd_dot input; yd_dot input; thetab output
function thetab = thB(xd_dot,yd_dot)

thetab = atan2(yd_dot, xd_dot);


end

== matlab function controllerJohnny/LinearlizationCTR/Trajectory ==
  data: t input; xd output; yd output; xd_dot output; yd_dot output; xd_ddot output; yd_ddot output
function [xd, yd, xd_dot, yd_dot, xd_ddot, yd_ddot] = traj(t)
 
R = 6;
w = 0.4;

xd = R*cos(w*t);
yd = R*sin(w*t);

xd_dot = -R*w*sin(w*t);
yd_dot =  R*w*cos(w*t);

xd_ddot = -R*w^2*cos(w*t);
yd_ddot = -R*w^2*sin(w*t);
end

%{
    T = mod(t,8);
    v = 2;

    if T < 2
                xd = v*T; yd = 0;
                xd_dot = v; yd_dot = 0;
            elseif T < 4
                xd = v*2; yd = v*(T-2);
                xd_dot = 0; yd_dot = v;
            elseif T < 6
                xd = v*(6-T); yd = v*2;
                xd_dot = -v; yd_dot = 0;
            else
                xd = 0; yd = v*(8-T);
                xd_dot = 0; yd_dot = -v;
    end

            xd_ddot = 0;
            yd_ddot = 0;
    end

%}

%{
% Square parameters
L = 18;        % side length [m]
v = 2;      % linear speed [m/s]
T = L / v;    % time per side

% Make trajectory periodic
t = mod(t, 4*T);

% Initialize outputs (VERY IMPORTANT for Simulink)
xd = 0; yd = 0;
xd_dot = 0; yd_dot = 0;
xd_ddot = 0; yd_ddot = 0;

% ---- Side 1: move right ----
if t < T
    xd = v*t;
    yd = 0;
    xd_dot = v;
    yd_dot = 0;

% ---- Side 2: move up ----
elseif t < 2*T
    xd = L;
    yd = v*(t - T);
    xd_dot = 0;
    yd_dot = v;

% ---- Side 3: move left ----
elseif t < 3*T
    xd = L - v*(t - 2*T);
    yd = L;
    xd_dot = -v;
    yd_dot = 0;

% ---- Side 4: move down ----
else
    xd = 0;
    yd = L - v*(t - 3*T);
    xd_dot = 0;
    yd_dot = -v;
end
end 
%}

%{
% ===== Parameters =====
v = 0.6;              % nominal speed
T1 = 5;               % straight
T2 = 6;               % curve
T3 = 8;               % long straight
T4 = 6;               % second curve
T5 = 5;               % final straight
Tstop = 4;            % stop time

% Cumulative times
t1 = T1;
t2 = t1 + T2;
t3 = t2 + T3;
t4 = t3 + T4;
t5 = t4 + T5;
tf = t5 + Tstop;

% Saturate time (robot stops at final point)
t = min(t, tf);

% Initialize outputs (IMPORTANT)
xd = 0; yd = 0;
xd_dot = 0; yd_dot = 0;
xd_ddot = 0; yd_ddot = 0;

% ===== Phase 1: straight =====
if t < t1
    xd = v*t;
    yd = 0;
    xd_dot = v;

% ===== Phase 2: smooth curve (avoid obstacle) =====
elseif t < t2
    tau = (t - t1)/T2;
    xd = v*t1 + v*T2*tau;
    yd = 2*sin(pi*tau);
    xd_dot = v;
    yd_dot = 2*pi*cos(pi*tau)/T2;

% ===== Phase 3: long straight =====
elseif t < t3
    xd = v*t;
    yd = 2;
    xd_dot = v;

% ===== Phase 4: second curve =====
elseif t < t4
    tau = (t - t3)/T4;
    xd = v*t3 + v*T4*tau;
    yd = 2 + 2*sin(pi*tau);
    xd_dot = v;
    yd_dot = 2*pi*cos(pi*tau)/T4;

% ===== Phase 5: final straight =====
elseif t < t5
    xd = v*t;
    yd = 4;
    xd_dot = v;

% ===== Phase 6: STOP =====
else
    xd = v*t5;
    yd = 4;
    xd_dot = 0;
    yd_dot = 0;
end
end
%}

== matlab function controllerJohnny/Output-error feedbackCTR3/Trajectory1 ==
  data: t input; xd output; yd output; xd_dot output; yd_dot output; xd_ddot output; yd_ddot output
function [xd, yd, xd_dot, yd_dot, xd_ddot, yd_ddot] = traj(t)
%{
R = 6;
w = 0.4;

xd = R*cos(w*t);
yd = R*sin(w*t);

xd_dot = -R*w*sin(w*t);
yd_dot =  R*w*cos(w*t);

xd_ddot = -R*w^2*cos(w*t);
yd_ddot = -R*w^2*sin(w*t);
end

%}
    T = mod(t,8);
    v = 2;

    if T < 2
                xd = v*T; yd = 0;
                xd_dot = v; yd_dot = 0;
            elseif T < 4
                xd = v*2; yd = v*(T-2);
                xd_dot = 0; yd_dot = v;
            elseif T < 6
                xd = v*(6-T); yd = v*2;
                xd_dot = -v; yd_dot = 0;
            else
                xd = 0; yd = v*(8-T);
                xd_dot = 0; yd_dot = -v;
    end

            xd_ddot = 0;
            yd_ddot = 0;
    end



%{
% Square parameters
L = 24;        % side length [m]
v = 6;      % linear speed [m/s]
T = L / v;    % time per side

% Make trajectory periodic
t = mod(t, 4*T);

% Initialize outputs (VERY IMPORTANT for Simulink)
xd = 0; yd = 0;
xd_dot = 0; yd_dot = 0;
xd_ddot = 0; yd_ddot = 0;

% ---- Side 1: move right ----
if t < T
    xd = v*t;
    yd = 0;
    xd_dot = v;
    yd_dot = 0;

% ---- Side 2: move up ----
elseif t < 2*T
    xd = L;
    yd = v*(t - T);
    xd_dot = 0;
    yd_dot = v;

% ---- Side 3: move left ----
elseif t < 3*T
    xd = L - v*(t - 2*T);
    yd = L;
    xd_dot = -v;
    yd_dot = 0;

% ---- Side 4: move down ----
else
    xd = 0;
    yd = L - v*(t - 3*T);
    xd_dot = 0;
    yd_dot = -v;
end
end 
%}


   % obstacle_traj
%{

% ===== Parameters =====
v = 0.6;              % nominal speed
T1 = 5;               % straight
T2 = 6;               % curve
T3 = 8;               % long straight
T4 = 6;               % second curve
T5 = 5;               % final straight
Tstop = 4;            % stop time

% Cumulative times
t1 = T1;
t2 = t1 + T2;
t3 = t2 + T3;
t4 = t3 + T4;
t5 = t4 + T5;
tf = t5 + Tstop;

% Saturate time (robot stops at final point)
t = min(t, tf);

% Initialize outputs (IMPORTANT)
xd = 0; yd = 0;
xd_dot = 0; yd_dot = 0;
xd_ddot = 0; yd_ddot = 0;

% ===== Phase 1: straight =====
if t < t1
    xd = v*t;
    yd = 0;
    xd_dot = v;

% ===== Phase 2: smooth curve (avoid obstacle) =====
elseif t < t2
    tau = (t - t1)/T2;
    xd = v*t1 + v*T2*tau;
    yd = 2*sin(pi*tau);
    xd_dot = v;
    yd_dot = 2*pi*cos(pi*tau)/T2;

% ===== Phase 3: long straight =====
elseif t < t3
    xd = v*t;
    yd = 2;
    xd_dot = v;

% ===== Phase 4: second curve =====
elseif t < t4
    tau = (t - t3)/T4;
    xd = v*t3 + v*T4*tau;
    yd = 2 + 2*sin(pi*tau);
    xd_dot = v;
    yd_dot = 2*pi*cos(pi*tau)/T4;

% ===== Phase 5: final straight =====
elseif t < t5
    xd = v*t;
    yd = 4;
    xd_dot = v;

% ===== Phase 6: STOP =====
else
    xd = v*t5;
    yd = 4;
    xd_dot = 0;
    yd_dot = 0;
end
end
%}

== matlab function controllerJohnny/LinearlizationCTR/Flatness ==
  data: xd_dot input; vd output; thetad output; omegad output; yd_dot input; xd_ddot input; yd_ddot input
function [vd, thetad, omegad] = flatness(xd_dot, yd_dot, xd_ddot, yd_ddot)

vd = sqrt(xd_dot^2 + yd_dot^2);
thetad = atan2(yd_dot, xd_dot);
omegad = (xd_dot*yd_ddot - yd_dot*xd_ddot)/max(vd^2,1e-3);
end

== matlab function controllerJohnny/Output-error feedbackCTR3/Subsystem/U2 ==
  data: x input; y input; theta input; y1 output; y2 output; b output
function [y1, y2,b] = inversTransform(x,y,theta)
b = 0.5;
y1 = x + b * cos(theta);
y2 = y + b * sin(theta);

end

== matlab function controllerJohnny/LinearlizationCTR/Rotation1 ==
  data: ex input; e output; ey input; etheta input; theta input
function e = error_transform(ex, ey, etheta, theta)

e1 =  ex*cos(theta) + ey*sin(theta);
e2 = -ex*sin(theta) + ey*cos(theta);
e3 = etheta;

e = [e1 e2 e3];
end

== matlab function controllerJohnny/LinearlizationCTR/Gians ==
  data: vd input; k1 output; k2 output; k3 output; wdes input; xi output; a output
function [k1, k2, k3,xi,a] = gain_scheduler(vd, wdes)


%{
% good value or the sequare 
xi = 0.7;
a  = 10;
%}
xi = 0.7;
a  = 1;

k1 = 2*xi*a;
k3 = 2*xi*a;

% avoid division by zero
eps = 1e-3;
k2 = (a^2 - wdes^2) / max(vd, eps);
end

== matlab function controllerJohnny/LinearlizationCTR/U ==
  data: k1 input; k2 input; k3 input; e input; u1 output; u2 output; e3 output
function [u1, u2,e3] = linear_controller(k1, k2, k3 ,e)

u1 = -k1 * e(1);
u2 = -k2 * e(2) - k3 * e(3);
e3 =e(3);

end
